simulink model "A2_1_P_velocity"  (Simulink 7.4)
settings: Solver=FixedStepDiscrete  StartTime=0.0  StopTime=5  RelTol=1e-3
undefined symbols (not defined in the file): Kp
libraries: DCmotor_library x1
settings Model: Creator=Natalia  LastModifiedBy=ma
settings DebuggingCC: StrictBusMsg=ErrorLevel1
settings HardwareCC: ProdIntDivRoundTo=Zero  ProdEndianess=LittleEndian  ProdHWDeviceType=Generic->32-bit x86 compatible
settings RTWCC: ProcessScript=grt_make_rtw_hook  RTWCompilerOptimization=On
settings CodeAppCC: MaxIdLength=95  CustomSymbolStrType=$N$R$M_T
settings GRTTargetCC: CombineOutputUpdateFcns=on

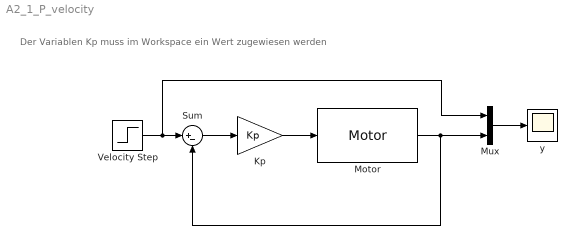
== system A2_1_P_velocity ==
  note: Der Variablen Kp
      | muss im Workspace ein
      | Wert zugewiesen werden
  Kp : Gain  Gain=Kp
  Motor : DCmotor_library/Motor  motoridinput=1  name_signal=Velocity  ts=10
  Mux : Mux  Inputs=2
  Sum : Sum  Inputs=|+-
  Velocity Step : Step  After=47.75  SampleTime=0
  y : Scope
      settings: YMax=50
  wires:
  Velocity Step/1 -> Mux/1, Sum/1
  Motor/1 -> Mux/2, Sum/2
  Sum/1 -> Kp/1
  Kp/1 -> Motor/1
  Mux/1 -> y/1
